simulink model "button_to_force_mocap"  (R2023b)
settings: Solver=FixedStepAuto  StartTime=0.0  StopTime=inf  RelTol=1e-3  EnableMultiTasking=on
model workspace (MAT data in the model file):
  G = 2001
undefined symbols (not defined in the file): c_t, f_max, f_min, Kd, Kp, M, W
libraries: rpi_blkst x3, dspfdesign x3, robotcorelib x1
settings Model: ExtModeTrigDuration=2  Creator=yabde  LastModifiedBy=yabde
settings SolverCC: PositivePriorityOrder=on
settings OptimizationCC: EnhancedBackFolding=on  PassReuseOutputArgsAs=Individual arguments  ZeroExternalMemoryAtStartup=off  ZeroInternalMemoryAtStartup=off  MaxStackSize=64  OptimizeBlockOrder=speed  DifferentSizesBufferReuse=on  OptimizationCustomize=off  EfficientTunableParamExpr=on
settings DebuggingCC: ParameterTunabilityLossMsg=error
settings HardwareCC: ProdBitPerLong=64  ProdLargestAtomicInteger=LongLong  ProdLargestAtomicFloat=Double  ProdLongLongMode=on  ProdHWDeviceType=ARM Compatible->ARM 64-bit (LP64)
settings RTWCC: Description=Embedded Coder  SystemTargetFile=ert.tlc  HardwareBoard=Raspberry Pi (64bit)  TLCOptions="-aInlineSetEventsForThisBaseRateFcn=TLC_FALSE -aSuppressMultiTaskScheduler=TLC_FALSE  -aRateBasedStepFcn=0"  TemplateMakefile=ert_default_tmf  Toolchain=GNU GCC Embedded Linux  BuildConfiguration=Faster Runs
settings CodeAppCC: ForceParamTrailComments=on  IgnoreCustomStorageClasses=off  OperatorAnnotations=on  SimulinkDataObjDesc=on  SFDataObjDesc=on  InsertBlockDesc=on
settings ERTTargetCC: SupportVariableSizeSignals=on  ExtModeTransport=2  ExtModeStaticAlloc=on  ExtModeMexFile=ext_xcp  ExtModeIntrfLevel=Level2 - Open

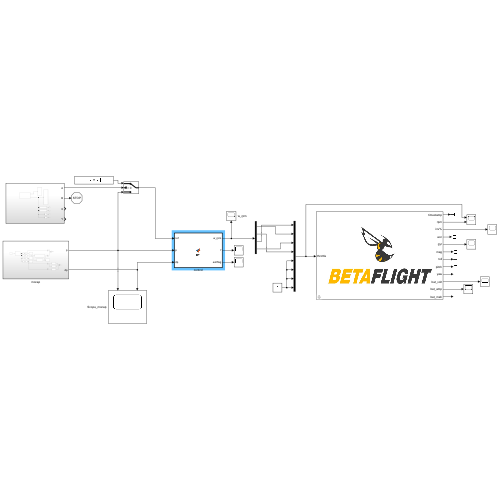
[thumbnail: Simulink's stored preview of the top-level diagram]
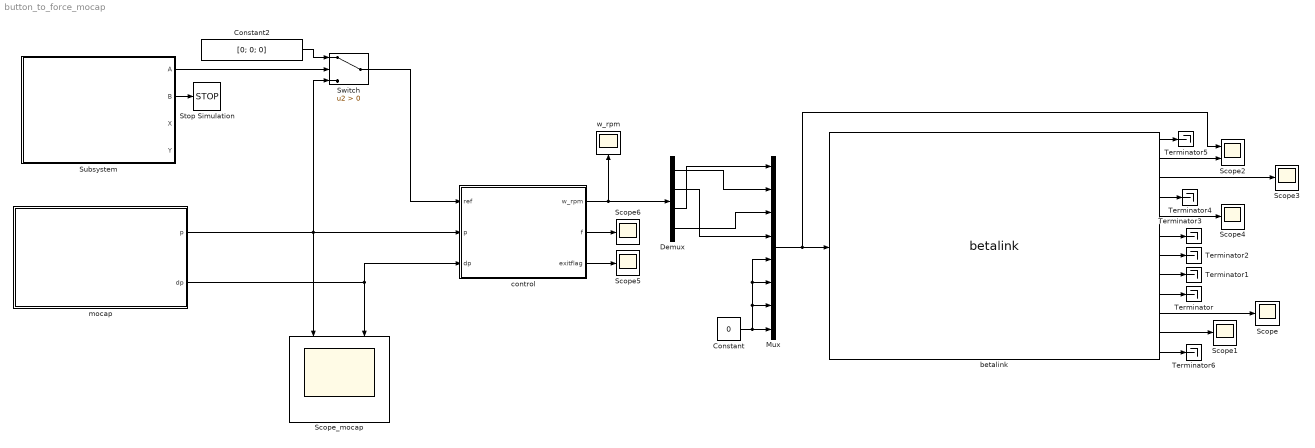
== system button_to_force_mocap ==
  Constant : Constant  Value=0
  Constant2 : Constant  Value=[0; 0; 0]
  Demux : Demux
  Mux : Mux  Inputs=8
  Scope{,1,3..6} (6 alike) : Scope
  Scope2 : Scope  NumInputPorts=2
  Scope_mocap : Scope  NumInputPorts=2
  Stop Simulation : Stop
  Subsystem : Subsystem
  Switch : Switch  Criteria=u2 > Threshold  SaturateOnIntegerOverflow=off  InputSameDT=off
  Terminator{,1..6} (7 alike) : Terminator
  betalink : rpi_blkst/betalink  rpi_mask_usb_serial_number=1042260556  rpi_mask_Ts=0.01
      settings: SourceProductName=RPI Blockset
  control : MATLAB Function  TreatAsAtomicUnit=on
  mocap : Subsystem
  w_rpm : Scope
  wires:
  Mux/1 -> betalink/1, Scope2/1
  Constant/1 -> Mux/5, Mux/6, Mux/7, Mux/8
  betalink/10 -> Scope/1
  betalink/11 -> Scope1/1
  betalink/2 -> Scope2/2
  betalink/3 -> Scope3/1
  betalink/5 -> Scope4/1
  betalink/9 -> Terminator/1
  betalink/8 -> Terminator1/1
  betalink/7 -> Terminator2/1
  betalink/6 -> Terminator3/1
  betalink/4 -> Terminator4/1
  betalink/12 -> Terminator6/1
  betalink/1 -> Terminator5/1
  control/1(w_rpm) -> w_rpm/1, Demux/1
  Demux/1 -> Mux/2
  Demux/2 -> Mux/4
  Demux/3 -> Mux/1
  Demux/4 -> Mux/3
  mocap/2(dp) -> Scope_mocap/2, control/3(dp)
  control/2(f) -> Scope6/1
  control/3(exitflag) -> Scope5/1
  Subsystem/2(B) -> Stop Simulation/1
  Subsystem/1(A) -> Switch/2
  Switch/1 -> control/1(ref)
  mocap/1(p) -> Switch/3, control/2(p), Scope_mocap/1
  Constant2/1 -> Switch/1

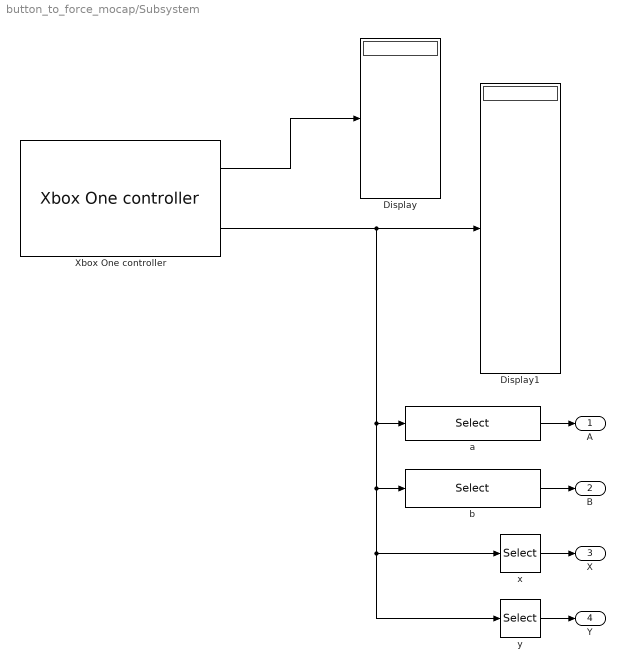
== system button_to_force_mocap/Subsystem ==
  Display : Display
  Display1 : Display
  Xbox One controller : rpi_blkst/Xbox One controller  rpi_mask_ID=0  rpi_mask_Ts=0.01
      settings: SourceProductName=RPI Blockset
  a : Selector  IndexOptions=Index vector (dialog)  Indices=1  OutputSizes=1  RuntimeRangeChecks=on
  b : Selector  IndexOptions=Index vector (dialog)  Indices=2  OutputSizes=1  RuntimeRangeChecks=on
  x : Selector  IndexOptions=Index vector (dialog)  Indices=4  OutputSizes=1  RuntimeRangeChecks=on
  y : Selector  IndexOptions=Index vector (dialog)  Indices=5  OutputSizes=1  RuntimeRangeChecks=on
  A : Outport
  B : Outport  Port=2
  X : Outport  Port=3
  Y : Outport  Port=4
  wires:
  Xbox One controller/1 -> Display/1
  Xbox One controller/2 -> y/1, x/1, b/1, a/1, Display1/1
  y/1 -> Y/1
  x/1 -> X/1
  a/1 -> A/1
  b/1 -> B/1

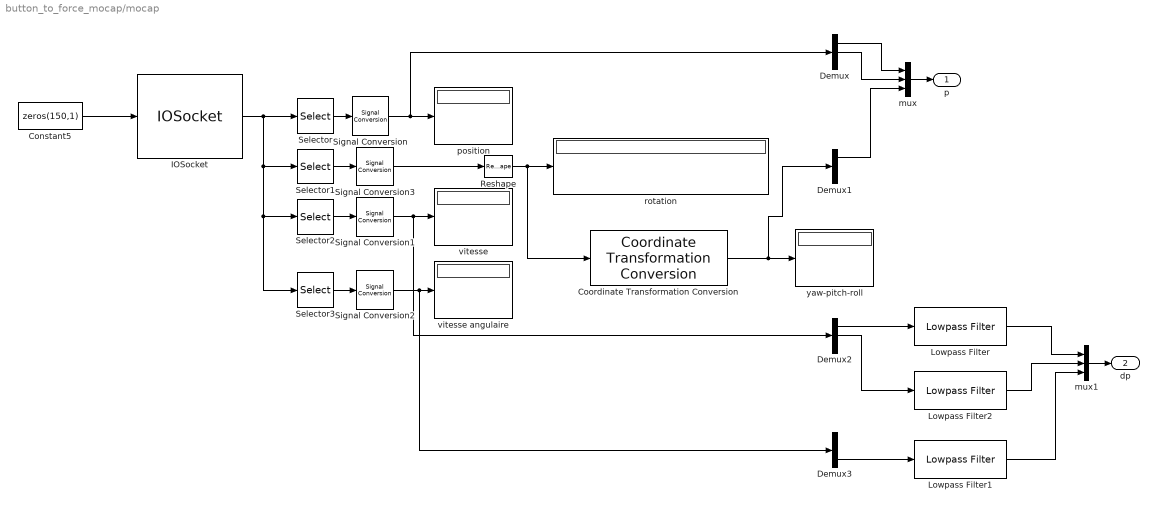
== system button_to_force_mocap/mocap ==
  Constant5 : Constant  Value=zeros(150,1)
  Coordinate Transformation Conversion : robotcorelib/Coordinate Transformation Conversion  InputRepresentation=Rotation Matrix  InputEulerSequence=ZYX  ShowTrVecInputPort=on  OutputRepresentation=Euler Angles  OutputEulerSequence=ZYX  ShowTrVecOutputPort=on  SimulateUsing=Interpreted execution
  Demux{,1..3} (4 alike) : Demux  Outputs=3
  IOSocket : rpi_blkst/IOSocket  rpi_mask_Ts=0.01  rpi_mask_ip1=192  rpi_mask_ip2=168  rpi_mask_ip3=0  rpi_mask_ip4=13  rpi_mask_port=31415
      settings: SourceProductName=RPI Blockset
  Lowpass Filter : dspfdesign/Lowpass Filter  FilterType=IIR  DesignForMinimumOrder=on  FilterOrder=50  PassbandFrequency=6  StopbandFrequency=15  PassbandRipple=0.2  StopbandAttenuation=40  SampleRateMode=Specify on dialog  SampleRate=100  SimulateUsing=Interpreted execution  roundingMode=Floor  coeffsDataTypeStr=fixdt(1,16)
  Lowpass Filter1 : dspfdesign/Lowpass Filter  FilterType=IIR  DesignForMinimumOrder=on  FilterOrder=50  PassbandFrequency=6  StopbandFrequency=15  PassbandRipple=0.2  StopbandAttenuation=40  SampleRateMode=Specify on dialog  SampleRate=100  SimulateUsing=Interpreted execution  roundingMode=Floor  coeffsDataTypeStr=fixdt(1,16)
  Lowpass Filter2 : dspfdesign/Lowpass Filter  FilterType=IIR  DesignForMinimumOrder=on  FilterOrder=50  PassbandFrequency=6  StopbandFrequency=15  PassbandRipple=0.2  StopbandAttenuation=40  SampleRateMode=Specify on dialog  SampleRate=100  SimulateUsing=Interpreted execution  roundingMode=Floor  coeffsDataTypeStr=fixdt(1,16)
  Reshape : Reshape  OutputDimensionality=Customize  OutputDimensions=[3,3]
  Selector : Selector  IndexOptions=Index vector (dialog)  Indices=3:5  OutputSizes=1
  Selector1 : Selector  IndexOptions=Index vector (dialog)  Indices=6:14  OutputSizes=1
  Selector2 : Selector  IndexOptions=Index vector (dialog)  Indices=15:17  OutputSizes=1
  Selector3 : Selector  IndexOptions=Index vector (dialog)  Indices=18:20  OutputSizes=1
  Signal Conversion{,1..3} (4 alike) : SignalConversion  OverrideOpt=off
  mux : Mux  Inputs=3
  mux1 : Mux  Inputs=3
  position : Display
  rotation : Display
  vitesse : Display
  vitesse angulaire : Display
  yaw-pitch-roll : Display
  p : Outport
  dp : Outport  Port=2
  wires:
  Selector2/1 -> Signal Conversion1/1
  Signal Conversion1/1 -> Demux2/1, vitesse/1
  Signal Conversion2/1 -> Demux3/1, vitesse angulaire/1
  Selector/1 -> Signal Conversion/1
  Constant5/1 -> IOSocket/1
  Reshape/1 -> Coordinate Transformation Conversion/1, rotation/1
  IOSocket/1 -> Selector3/1, Selector2/1, Selector1/1, Selector/1
  Selector3/1 -> Signal Conversion2/1
  Signal Conversion/1 -> Demux/1, position/1
  Selector1/1 -> Signal Conversion3/1
  Signal Conversion3/1 -> Reshape/1
  Coordinate Transformation Conversion/1 -> Demux1/1, yaw-pitch-roll/1
  Demux/1 -> mux/1
  Demux/2 -> mux/2
  Demux1/1 -> mux/3
  mux/1 -> p/1
  mux1/1 -> dp/1
  Demux2/2 -> Lowpass Filter2/1
  Demux2/1 -> Lowpass Filter/1
  Demux3/3 -> Lowpass Filter1/1
  Lowpass Filter/1 -> mux1/1
  Lowpass Filter1/1 -> mux1/3
  Lowpass Filter2/1 -> mux1/2

== matlab function button_to_force_mocap/control ==
  data: ref input; w_rpm output size=4; f output; Kp parameter; Kd parameter; M parameter; c_t parameter; f_min parameter; f_max parameter; exitflag output; W parameter; p input; dp input
function [w_rpm,f,exitflag] = fcn(ref, Kp, Kd, M, c_t, f_min, f_max, W, p, dp)

ref = Kp * (ref - p); % - Kd * dp;

%% Formulation QP : min ||f||^2 s.t. W*f = tau and fmin <= f <= fmax
H = eye(4);
f_qp = zeros(4,1);

Aeq = W;
beq = ref;

f0 = W \ ref;

%% Résolution
options = optimoptions('quadprog', 'Display', 'off', 'Algorithm', 'active-set');
[f,~,exitflag,~] = quadprog(H, f_qp, [], [], Aeq, beq, f_min, f_max, f0, options);

f = min(max(f, f_min), f_max);

%% Conversion
w = sqrt(f ./ c_t);
w_rpm = (w * 30/pi);
